simulink model "s2dot2_demux"  (R2023b)
settings: Solver=VariableStepAuto  StartTime=0.0  StopTime=10.0  RelTol=1e-3
settings Model: Creator=lxj  LastModifiedBy=lxj

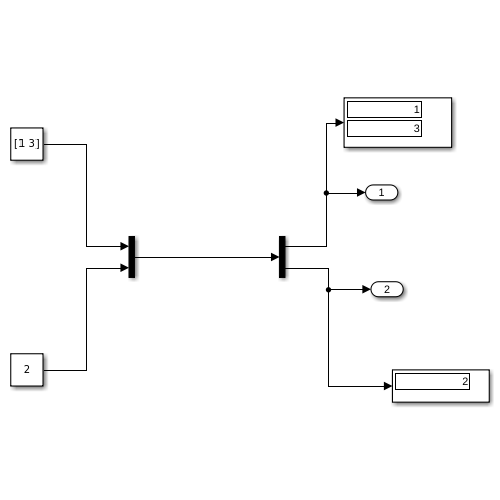
[thumbnail: Simulink's stored preview of the top-level diagram]
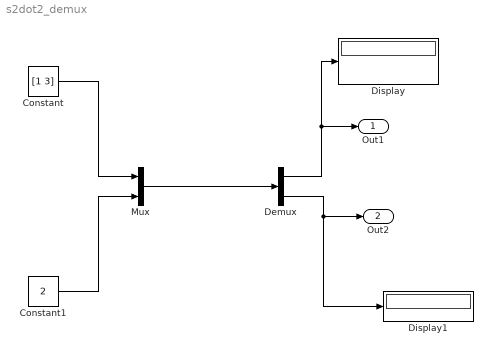
== system s2dot2_demux ==
  Constant : Constant  Value=[1 3]
  Constant1 : Constant  Value=2
  Demux : Demux  Outputs=2
  Display : Display
  Display1 : Display
  Mux : Mux  Inputs=2
  Out1 : Outport
  Out2 : Outport  Port=2
  wires:
  Mux/1 -> Demux/1
  Demux/1 -> Display/1, Out1/1
  Demux/2 -> Display1/1, Out2/1
  Constant1/1 -> Mux/2
  Constant/1 -> Mux/1
